simulink model "super"  (R2015a)
settings: Solver=ode3  StartTime=0.0  StopTime=24*3600  FixedStep=1  RelTol=1e-3
libraries: refrigeration x1
settings Model: CovSFcnEnable=off  Creator=avenger  LastModifiedBy=wbernalh
settings DataIOCC: LimitDataPoints=off
settings DebuggingCC: SolverPrmCheckMsg=warning

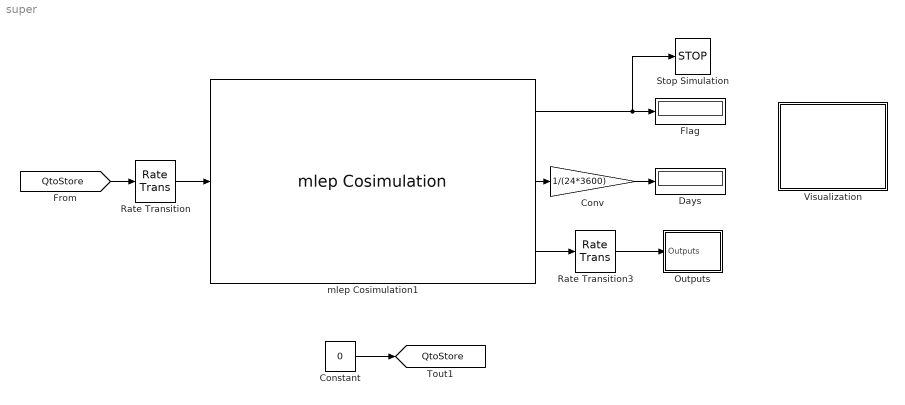
== system super ==
  Constant : Constant  Value=0
  Conv : Gain  Gain=1/(24*3600)
  Days : Display
  Flag : Display
  Outputs : Subsystem
  Rate Transition : RateTransition
  Rate Transition3 : RateTransition
  Stop Simulation : Stop
  Visualization : Subsystem
  mlep Cosimulation1 : refrigeration/mlep Cosimulation  progname='runenergyplus'  idf='super_noSi_noCa'  weather='USA_FL_Miami.Intl.AP.722020_TMY3'  timeout=2000  step=300  numinput=1  numoutput=4  bcvtbpath='/Users/wbernalh/Documents/git/refrigeration/RefrigerationLibrary/bcvtb'
  tag scope: QtoStore=global
  wires:
  mlep Cosimulation1/2 -> Conv/1
  mlep Cosimulation1/1 -> Stop Simulation/1, Flag/1
  mlep Cosimulation1/3 -> Rate Transition3/1
  Conv/1 -> Days/1
  Rate Transition3/1 -> Outputs/1(Outputs)
  [QtoStore] -> Rate Transition/1
  Rate Transition/1 -> mlep Cosimulation1/1
  Constant/1 -> [QtoStore]

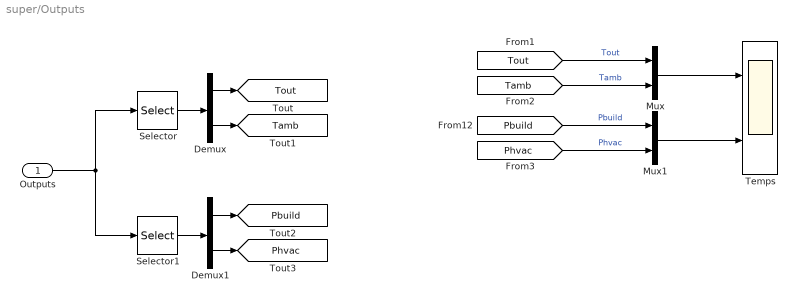
== system super/Outputs ==
  Outputs : Inport
  Demux : Demux  Outputs=2
  Demux1 : Demux  Outputs=2
  Mux : Mux  Inputs=2
  Mux1 : Mux  Inputs=2
  Selector : Selector  InputPortWidth=4  Indices=[1:2]
  Selector1 : Selector  InputPortWidth=4  Indices=[3:4]
  Temps : Scope  NumInputPorts=2
      settings: ShowLegends=on  TimeRange=90000  YMin=0~0  YMax=35~14000
  tag scope: Pbuild=global, Phvac=global, Tamb=global, Tout=global
  wires:
  [Tout] -> Mux/1  "Tout"
  [Tamb] -> Mux/2  "Tamb"
  Mux/1 -> Temps/1
  [Pbuild] -> Mux1/1  "Pbuild"
  Selector/1 -> Demux/1
  Demux/1 -> [Tout]
  Demux/2 -> [Tamb]
  Outputs/1 -> Selector1/1, Selector/1
  Selector1/1 -> Demux1/1
  Demux1/1 -> [Pbuild]
  Demux1/2 -> [Phvac]
  Mux1/1 -> Temps/2
  [Phvac] -> Mux1/2  "Phvac"

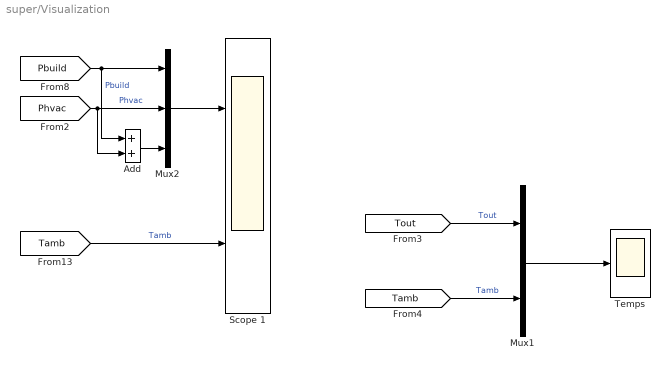
== system super/Visualization ==
  Add : Sum
  Mux1 : Mux  Inputs=2
  Mux2 : Mux  Inputs=3
  Scope 1 : Scope  NumInputPorts=2
      settings: ShowLegends=on  TimeRange=86400  YMin=-4e+06~-30  YMax=1.5e+06~25  SaveName=ScopeData4
  Temps : Scope
      settings: ShowLegends=on  TimeRange=90000  YMin=-40  YMax=40
  wires:
  Mux1/1 -> Temps/1
  [Tout] -> Mux1/1  "Tout"
  [Tamb] -> Mux1/2  "Tamb"
  [Pbuild] -> Add/1, Mux2/1  "Pbuild"
  [Tamb] -> Scope 1/2  "Tamb"
  Mux2/1 -> Scope 1/1
  [Phvac] -> Add/2, Mux2/2  "Phvac"
  Add/1 -> Mux2/3
